simulink model "Path_Planning_SFunc_Simulink"  (R2021a)
settings: Solver=VariableStepAuto  StartTime=0.0  StopTime=5  RelTol=1e-3
settings Model: Creator=WU  LastModifiedBy=WU

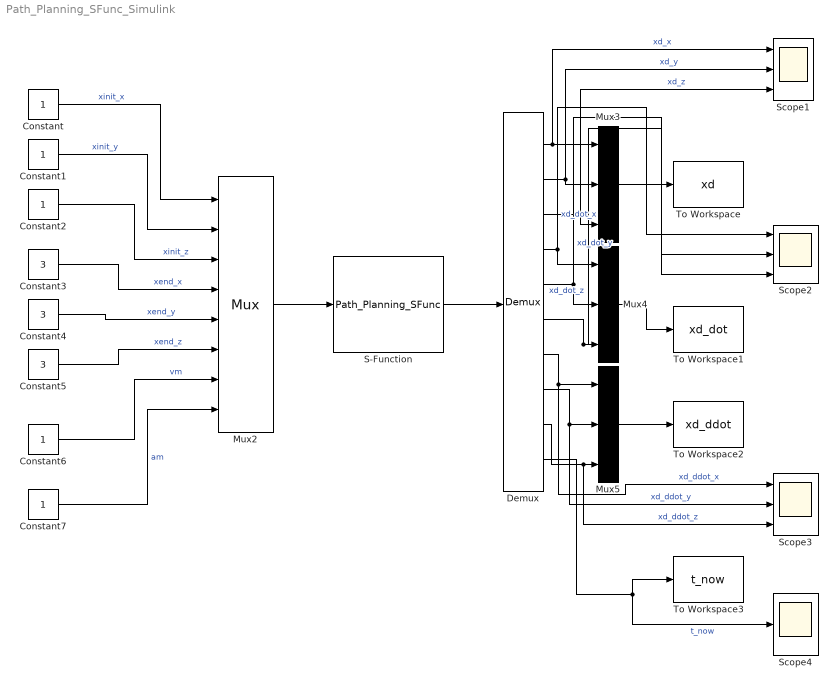
== system Path_Planning_SFunc_Simulink ==
  Constant : Constant  VectorParams1D=off
  Constant{1..2,6..7} (4 alike) : Constant
  Constant3 : Constant  Value=3
  Constant4 : Constant  Value=3
  Constant5 : Constant  Value=3
  Demux : Demux  Outputs=10
      settings: DisplayOption=none
  Mux2 : Mux  Inputs=8
  Mux3 : Mux  Inputs=3
  Mux4 : Mux  Inputs=3
  Mux5 : Mux  Inputs=3
  S-Function : S-Function  FunctionName=Path_Planning_SFunc  SFunctionDeploymentMode=off  EnableBusSupport=off
  Scope1 : Scope  NumInputPorts=3
  Scope2 : Scope  NumInputPorts=3
  Scope3 : Scope  NumInputPorts=3
  Scope4 : Scope
  To Workspace : ToWorkspace  VariableName=xd  SampleTime=-1
  To Workspace1 : ToWorkspace  VariableName=xd_dot  SampleTime=-1
  To Workspace2 : ToWorkspace  VariableName=xd_ddot  SampleTime=-1
  To Workspace3 : ToWorkspace  VariableName=t_now  SampleTime=-1
  wires:
  Constant/1 -> Mux2/1  "xinit_x"
  Constant2/1 -> Mux2/3  "xinit_z"
  Constant3/1 -> Mux2/4  "xend_x"
  Constant4/1 -> Mux2/5  "xend_y"
  Constant5/1 -> Mux2/6  "xend_z"
  Mux2/1 -> S-Function/1
  S-Function/1 -> Demux/1
  Demux/1 -> Scope1/1, Mux3/1  "xd_x"
  Demux/2 -> Mux3/2, Scope1/2  "xd_y"
  Demux/3 -> Mux3/3, Scope1/3  "xd_z"
  Mux3/1 -> To Workspace/1
  Demux/4 -> Mux4/1, Scope2/1  "xd_dot_x"
  Demux/6 -> Scope2/3, Mux4/3  "xd_dot_z"
  Demux/5 -> Mux4/2, Scope2/2  "xd_dot_y"
  Mux4/1 -> To Workspace1/1
  Demux/7 -> Scope3/1, Mux5/1  "xd_ddot_x"
  Demux/8 -> Scope3/2, Mux5/2  "xd_ddot_y"
  Demux/9 -> Scope3/3, Mux5/3  "xd_ddot_z"
  Mux5/1 -> To Workspace2/1
  Constant1/1 -> Mux2/2  "xinit_y"
  Constant6/1 -> Mux2/7  "vm"
  Constant7/1 -> Mux2/8  "am"
  Demux/10 -> To Workspace3/1, Scope4/1  "t_now"
